simulink model "Pendubot_PFL_LQR"  (R2025b)
settings: Solver=FixedStepAuto  StartTime=0.0  StopTime=Tsim  FixedStep=T  RelTol=1e-3
values from neighbouring files (symbols this model uses):
  Ad = Md(1:n, 1:n)    [k_LQR.m]
  Bd = Md(1:n, n+1)    [k_LQR.m]
  kalman = kalman_const(Ad, Bd)    [run_pendubot_simulink.m]
  noise_avg = 0.00    (= 0)    [run_pendubot_simulink.m]
  noise_std = 0.001    [run_pendubot_simulink.m]
  T = 1e-3    (= 0.001)    [kalman_const.m]    (also in pendubot_dynamics.m = 0.1; run_pendubot_simulink.m)
  X0 = [-90*pi/180; 0*pi/180; 0; 0]    [run_pendubot_simulink.m]
  xF = [pi/2; 0; 0; 0]    [run_pendubot_simulink.m]
undefined symbols (not defined in the file or in its folder): K
settings Model: NumberOfSteps=5  Creator=katiebyl  LastModifiedBy=24573

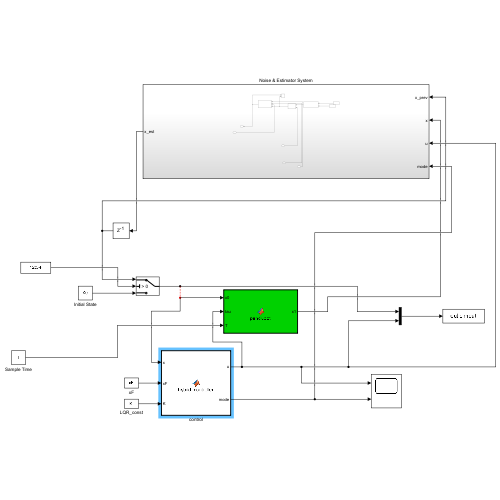
[thumbnail: Simulink's stored preview of the top-level diagram]
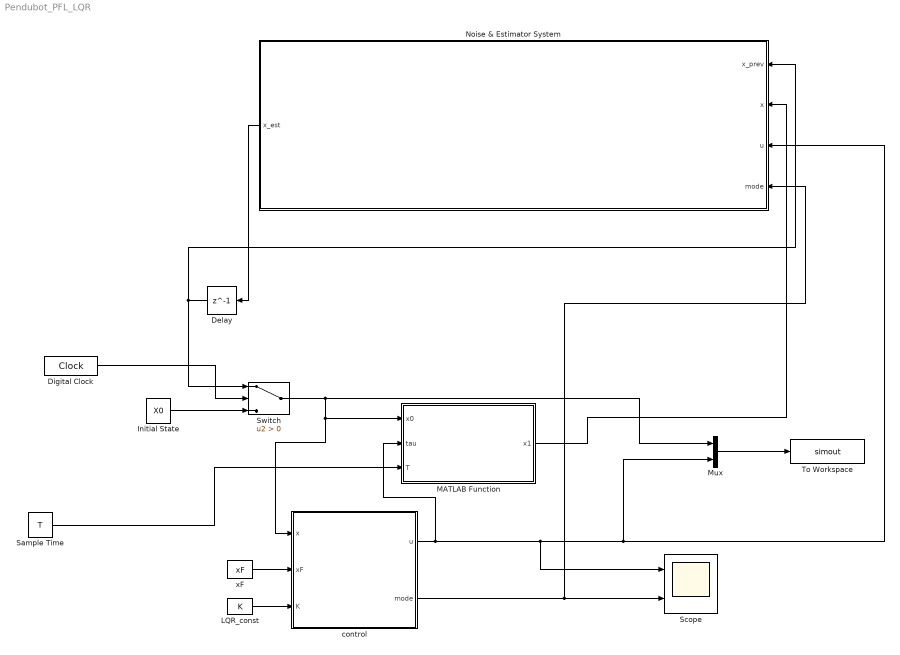
== system Pendubot_PFL_LQR ==
  Delay : Delay  DelayLength=1  InitialCondition=X0
  Digital Clock : DigitalClock  SampleTime=T
  Initial State : Constant  Value=X0
  LQR_const : Constant  Value=K
  MATLAB Function : MATLAB Function  TreatAsAtomicUnit=on
  Mux : Mux  Inputs=2
  Noise & Estimator System : Subsystem
  Sample Time : Constant  Value=T
  Scope : Scope  NumInputPorts=2
      settings: ActiveDisplayYMinimum=-17.41319411427747  ActiveDisplayYMaximum=11.909236160040471
  Switch : Switch  Criteria=u2 > Threshold  SaturateOnIntegerOverflow=off  InputSameDT=off
  To Workspace : ToWorkspace  VariableName=simout  SaveFormat=Timeseries  SampleTime=-1
  control : MATLAB Function  TreatAsAtomicUnit=on
  xF : Constant  Value=xF
  wires:
  Sample Time/1 -> MATLAB Function/3(T)
  Initial State/1 -> Switch/3
  Delay/1 -> Switch/1, Noise & Estimator System/1(x_prev)
  Digital Clock/1 -> Switch/2
  Switch/1 -> MATLAB Function/1(x0), control/1(x), Mux/1
  Mux/1 -> To Workspace/1
  LQR_const/1 -> control/3(K)
  control/1(u) -> Noise & Estimator System/3(u), Mux/2, Scope/1, MATLAB Function/2(tau)
  control/2(mode) -> Scope/2, Noise & Estimator System/4(mode)
  xF/1 -> control/2(xF)
  MATLAB Function/1(x1) -> Noise & Estimator System/2(x)
  Noise & Estimator System/1(x_est) -> Delay/1

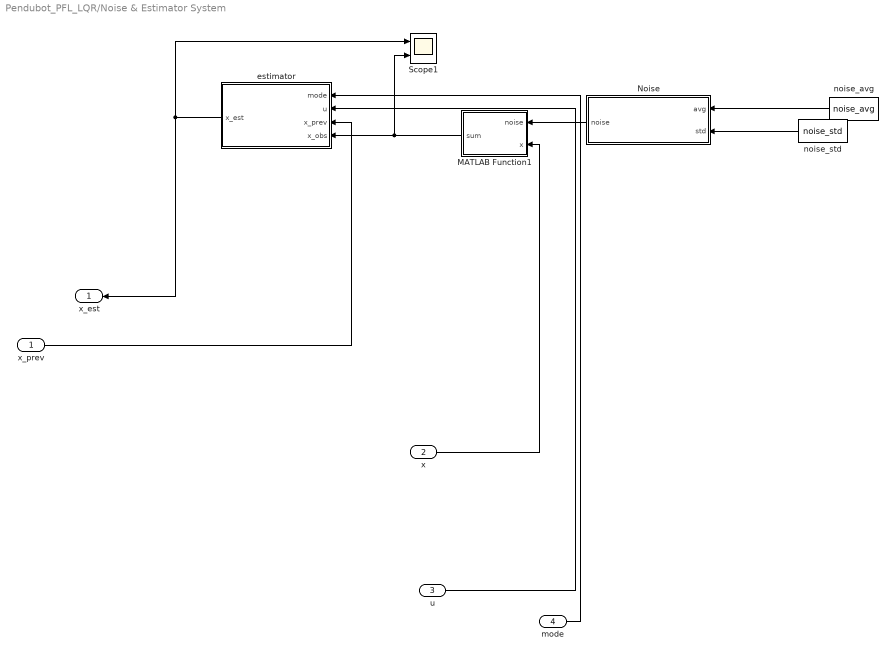
== system Pendubot_PFL_LQR/Noise & Estimator System ==
  x_prev : Inport
  x : Inport  Port=2
  u : Inport  Port=3
  mode : Inport  Port=4
  MATLAB Function1 : MATLAB Function  TreatAsAtomicUnit=on
  Noise : MATLAB Function  TreatAsAtomicUnit=on
  Scope1 : Scope  NumInputPorts=2
      settings: ActiveDisplayYMinimum=-1.7756523762872714E+82  ActiveDisplayYMaximum=9.74779643301642E+81
  estimator : Subsystem
  noise_avg : Constant  Value=noise_avg
  noise_std : Constant  Value=noise_std
  x_est : Outport
  wires:
  noise_avg/1 -> Noise/1(avg)
  MATLAB Function1/1(sum) -> Scope1/2, estimator/4(x_obs)
  Noise/1(noise) -> MATLAB Function1/1(noise)
  estimator/1(x_est) -> x_est/1, Scope1/1
  noise_std/1 -> Noise/2(std)
  u/1 -> estimator/2(u)
  x/1 -> MATLAB Function1/2(x)
  mode/1 -> estimator/1(mode)
  x_prev/1 -> estimator/3(x_prev)

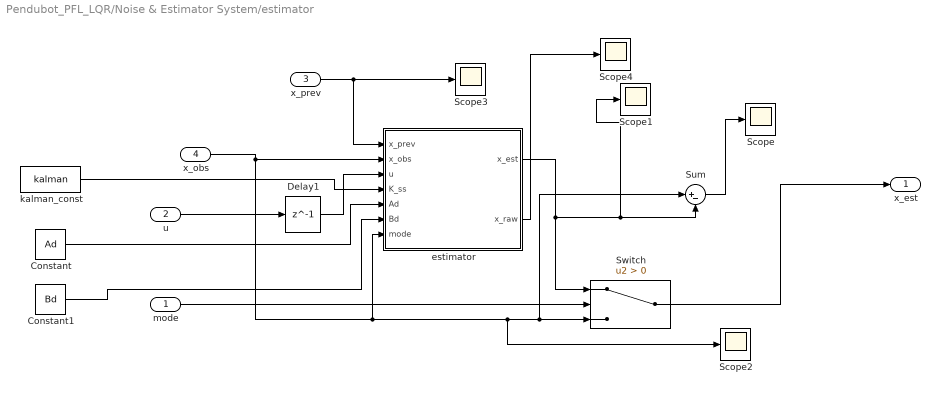
== system Pendubot_PFL_LQR/Noise & Estimator System/estimator ==
  mode : Inport
  u : Inport  Port=2
  x_prev : Inport  Port=3
  x_obs : Inport  Port=4
  Constant : Constant  Value=Ad
  Constant1 : Constant  Value=Bd
  Delay1 : Delay  DelayLength=1  InputProcessing=Columns as channels (frame based)
  Scope{,1..4} (5 alike) : Scope
      Scope settings: ActiveDisplayYMinimum=-67.083574034214379  ActiveDisplayYMaximum=133.24096460125318  DataLoggingVariableName=ScopeData2
      Scope1 settings: ActiveDisplayYMinimum=-173.46667177039649  ActiveDisplayYMaximum=114.21061141198169  DataLoggingVariableName=ScopeData3
      Scope2 settings: ActiveDisplayYMinimum=-3.2861865479866146  ActiveDisplayYMaximum=2.8575496039479709  DataLoggingVariableName=ScopeData4
      Scope3 settings: ActiveDisplayYMinimum=-44.377624701124269  ActiveDisplayYMaximum=47.375507788700126  DataLoggingVariableName=ScopeData5
      Scope4 settings: ActiveDisplayYMinimum=-31.974641520983919  ActiveDisplayYMaximum=15.329754631022812  DataLoggingVariableName=ScopeData6
  Sum : Sum  Inputs=|+-
  Switch : Switch  Criteria=u2 > Threshold  SaturateOnIntegerOverflow=off  InputSameDT=off
  estimator : MATLAB Function  TreatAsAtomicUnit=on
  kalman_const : Constant  Value=kalman
  x_est : Outport
  wires:
  mode/1 -> Switch/2
  Switch/1 -> x_est/1
  x_obs/1 -> estimator/2(x_obs), estimator/7(mode), Scope2/1, Sum/1, Switch/3
  estimator/1(x_est) -> Scope1/1, Sum/2, Switch/1
  u/1 -> Delay1/1
  Delay1/1 -> estimator/3(u)
  kalman_const/1 -> estimator/4(K_ss)
  Constant/1 -> estimator/5(Ad)
  Constant1/1 -> estimator/6(Bd)
  x_prev/1 -> Scope3/1, estimator/1(x_prev)
  Sum/1 -> Scope/1
  estimator/2(x_raw) -> Scope4/1

== matlab function Pendubot_PFL_LQR/control ==
  data: x input; xF input; K input; u output size=1; mode output
function [u, mode] = hybrid_controller(x, xF, K)
    u_max = 12;
    uF=0; kp = 4450;kd = 180;
    persistent lqr_engaged;
    if isempty(lqr_engaged)
        lqr_engaged = false;
    end
    % 1. Calculate Error
    error = x(1:4) - xF(1:4);
    
    % 2. Define Switching Condition
    e_pos = atan2(sin(error(1:2)), cos(error(1:2)));
    pos_err = norm(e_pos);
    e_vel = error(3:4);
    vel_err = norm(e_vel);

    %disp(error)
    if ((pos_err >= 0.8) || (vel_err >= 20.0)) && (lqr_engaged == false)
        % --- SWING UP MODE (Trajectory Playback) ---
        mode = 0;
        u = pendubot_pfl_controller(x(1:4), xF(1), xF(3), uF, kp, kd);
        %disp('PFL Activated');
        % disp(mode);
    else
        lqr_engaged = true;
        % --- LQR MODE ---
        mode = 1;
        x_error = [e_pos; e_vel];
        x_error = x_error(1:4, 1);
        K= K';
        u = -K(1,1:4)*x_error;
        u = u(1);
        % disp('LQR Activated');
    end
    
    % 3. Saturation (Physical Limits)
    u = max(min(u, u_max), -u_max);
    % disp(mode);
end


% --- PFL Helper: Calculates dynamics assuming q1_ddot = v ---
function dx = pfl_virtual_dynamics(x, v)
    % Unpack
    q1 = x(1); q2 = x(2); dq1 = x(3); dq2 = x(4);
    
    % Get Matrices
    [D, H, Phi] = get_matrices(x);
    d21 = D(2,1); d22 = D(2,2);
    h2 = H(2); phi2 = Phi(2);
    
    % If we force ddq1 = v, what happens to ddq2?
    % Equation 2: d21*v + d22*ddq2 + h2 + phi2 = 0
    % ddq2 = -inv(d22) * (d21*v + h2 + phi2)
    
    ddq2 = -(d21*v + h2 + phi2) / d22;
    
    dx = [dq1; dq2; v; ddq2];
end

% --- PFL Helper: Calculates Torque to achieve q1_ddot = v ---
function tau = inverse_dynamics_pfl(x, v)
    % Unpack
    % q1 = x(1); q2 = x(2); dq1 = x(3); dq2 = x(4);
    
    [D, H, Phi] = get_matrices(x);
    d11 = D(1,1); d12 = D(1,2);
    d21 = D(2,1); d22 = D(2,2);
    h1 = H(1); h2 = H(2);
    phi1 = Phi(1); phi2 = Phi(2);
    
    % From PFL derivation (Collocated Linearization):
    % tau = M_bar * v + N_bar
    
    % M_bar = d11 - d12*inv(d22)*d21
    m_bar = d11 - (d12 * d21 / d22);
    
    % N_bar = (h1 + phi1) - d12*inv(d22)*(h2 + phi2)
    n_bar = (h1 + phi1) - (d12 / d22) * (h2 + phi2);
    
    tau = m_bar * v + n_bar;
end

% --- Standard Matrices Helper ---
function [D, H, Phi] = get_matrices(x)
    q1 = x(1); q2 = x(2); dq1 = x(3); dq2 = x(4);
    
    g   = 9.81;
    Th1 = 3.08e-2; Th2 = 1.06e-2; Th3 = 9.5e-3;
    Th4 = 2.087e-1; Th5 = 6.3e-2;
    
    c2 = cos(q2); s2 = sin(q2);
    c1 = cos(q1); c12 = cos(q1+q2);

    D = [Th1 + Th2 + 2*Th3*c2,  Th2 + Th3*c2;
         Th2 + Th3*c2,          Th2];
     
    h_term = Th3 * s2;
    H = [-h_term * dq2 * (2*dq1 + dq2);
          h_term * dq1^2];
      
    Phi = [Th4*g*c1 + Th5*g*c12;
           Th5*g*c12];
end

%%pfl

function tau = pendubot_pfl_controller(x, q1d, dq1d, ddq1d, kp, kd)

% x = [q1;q2;dq1;dq2]
q1  = x(1);  q2  = x(2);
dq1 = x(3);  dq2 = x(4);

% Parameters (must match pendubot_dynamics.m)
g  = 9.8;
Th1 = 3.08e-2;
Th2 = 1.06e-2;
Th3 = 9.5e-3;
Th4 = 2.087e-1;
Th5 = 6.3e-2;

cosq1 = cos(q1);
cosq2 = cos(q2);
sinq2 = sin(q2);
cosq1q2 = cos(q1+q2);

% Inertia terms (same as dynamics file)
d11 = Th1 + Th2 + 2*Th3*cosq2;
d12 = Th2 + Th3*cosq2;
d22 = Th2;

% Coriolis/centrifugal terms
h1 = -Th3*sinq2*dq2*(dq1+dq2);
h2 =  Th3*sinq2*dq1^2;

% Gravity terms
phi1 = Th4*g*cosq1 + Th5*g*cosq1q2;
phi2 = Th5*g*cosq1q2;

% PFL scalars
Delta = d11 - (d12^2)/d22;
beta  = (h1 + phi1) - (d12/d22)*(h2 + phi2);

% Virtual input v to impose ddq1 = v
v = ddq1d - kd*(dq1 - dq1d) - kp*(q1 - q1d);

% Shoulder torque
tau = Delta*v + beta;

end

== matlab function Pendubot_PFL_LQR/MATLAB Function ==
  data: x0 input; x1 output; tau input; T input
function x1 = pendubot(x0, tau, T)

% function x1 = pendubot(x0)
%
% This function simulates the nonlinear dynamics of the
% pendubot on a discrete-time basis. 
%   input:  x0 is x(k)
%   output: x1 is x(k+1)
%
% The parameters are from the Pendubot manual, on the
% canvas page for "Final Project / Pendubot".
%
% Katie Byl, UCSB, ECE 238

% T = 1e-3; % Sample Time (s) - needs to match rest of model
g = 9.81; % gravity (m/(s^2))

Th1 = 3.08e-2;
Th2 = 1.06e-2;
Th3 = 9.5e-3;
Th4 = 2.087e-1;
Th5 = 6.3e-2;

q1 = x0(1); q2 = x0(2); % encoder angles, in radians
dq1 = x0(3); dq2 = x0(4); % angular velocities (rad/s)

cosq1 = cos(q1);
cosq2 = cos(q2); 
sinq2 = sin(q2);
cosq1q2 = cos(q1+q2);

d11 = Th1 + Th2 + 2 * Th3 * cosq2;
d12 = Th2 + Th3 * cosq2;
d22 = Th2;
D = [d11 d12; d12 d22];

h1 = -Th3 * sinq2 * dq2 * (dq1+dq2);
h2 = Th3 * sinq2 * dq1^2;
H = [h1; h2];

phi1 = Th4 * g * cosq1 + Th5 * g * cosq1q2;
phi2 = Th5 * g * cosq1q2;
Phi = [phi1; phi2];

Tau = [tau; 0]; % torque (N*m) applied to first link

%% Equation on motion, in matrix form, is:
%     D*d2q + H + Phi = [tau; 0] = Tau
%  (i.e., tau is applied at the FIRST link, for the pendubot)
%
%  Rearranging, we get:
%     D*d2q = Tau - H - Phi
%  which can be solved via the backslash:
%       d2q = D \ (Tau - H - Phi)

d2q = D \ (Tau - H - Phi);
dX = [x0(3:4); d2q]; % velocities and accelerations

% For "small T", we can use forward Euler to approximate
% the dynamics:

x1 = x0 + T*dX;  % forward Euler integration

%% End of function

== matlab function Pendubot_PFL_LQR/Noise & Estimator System/Noise ==
  data: avg input; noise output; std input
function noise = encoder_noise(avg, std)
    size = 4;
    noise_ = random('Normal', avg, std, size);
    noise__ = noise_(1,:);
    noise = noise__';
end

== matlab function Pendubot_PFL_LQR/Noise & Estimator System/MATLAB Function1 ==
  data: noise input; sum output; x input
function sum = add(noise, x)
    sum = x(1:4) + noise(1:4);

end

== matlab function Pendubot_PFL_LQR/Noise & Estimator System/estimator/estimator ==
  data: x_prev input; x_obs input; x_est output; u input; K_ss input; Ad input; Bd input; x_raw output; mode input
function [x_est, x_raw] = kalman_estimator(x_prev, x_obs, u, K_ss, Ad, Bd, mode)

    if mode == 1
        C = [1 0 0 0; 0 1 0 0]; 
        x_raw = Ad * x_prev + Bd * u;
        x_est = x_raw + K_ss * (x_obs(1:2) - C*(Ad*x_prev + Bd * u));
    else
        x_raw = [0;0;0;0];
        x_est = x_obs;
    end
end
